simulink model "model1"  (R2024b)
settings: Solver=VariableStepAuto  StartTime=0.0  StopTime=10.0  RelTol=1e-3
libraries: simulink x4
settings Model: Creator=mehmetcanevi  LastModifiedBy=mehmetcanevi

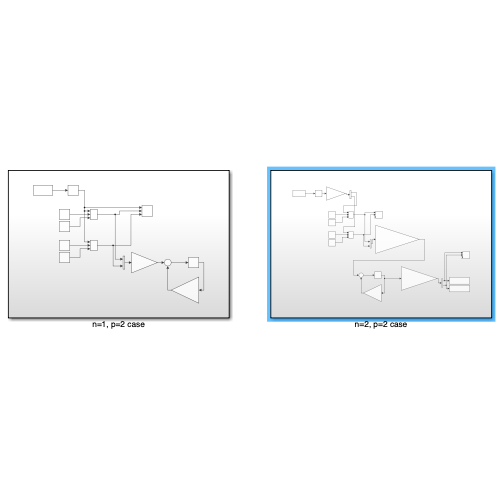
[thumbnail: Simulink's stored preview of the top-level diagram]
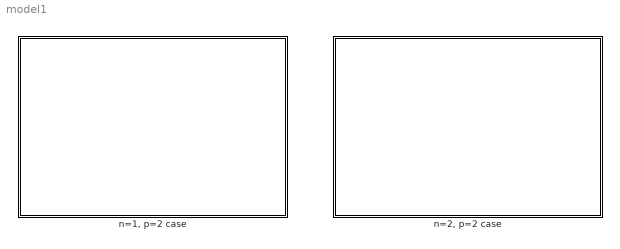
== system model1 ==
  "n=1, p=2 case" : Subsystem
  "n=2, p=2 case" : Subsystem

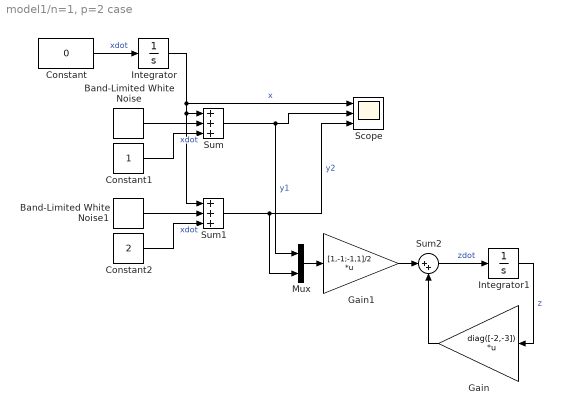
== system model1/n=1, p=2 case ==
  Band-Limited White Noise : simulink/Sources/Band-Limited White Noise  Cov=[0.001]  Ts=0.1  seed=[12345]
  Band-Limited White Noise1 : simulink/Sources/Band-Limited White Noise  Cov=[0.001]  Ts=0.1  seed=[12346]
  Constant : Constant  Value=0
  Constant1 : Constant
  Constant2 : Constant  Value=2
  Gain : Gain  Gain=diag([-2,-3])  Multiplication=Matrix(K*u)
  Gain1 : Gain  Gain=[1,-1;-1,1]/2  Multiplication=Matrix(K*u)
  Integrator : Integrator  InitialCondition=5
  Integrator1 : Integrator  InitialCondition=5
  Mux : Mux  Inputs=2
  Scope : Scope  NumInputPorts=3
  Sum : Sum  Inputs=+++
  Sum1 : Sum  Inputs=+++
  Sum2 : Sum  Inputs=|++
  wires:
  Sum2/1 -> Integrator1/1  "zdot"
  Constant1/1 -> Sum/3  "xdot"
  Band-Limited White Noise1/1 -> Sum1/2
  Integrator1/1 -> Gain/1  "z"
  Gain/1 -> Sum2/2
  Constant/1 -> Integrator/1  "xdot"
  Band-Limited White Noise/1 -> Sum/2
  Constant2/1 -> Sum1/3  "xdot"
  Integrator/1 -> Sum1/1, Sum/1, Scope/1  "x"
  Mux/1 -> Gain1/1
  Sum/1 -> Mux/1, Scope/2  "y1"
  Gain1/1 -> Sum2/1
  Sum1/1 -> Mux/2, Scope/3  "y2"

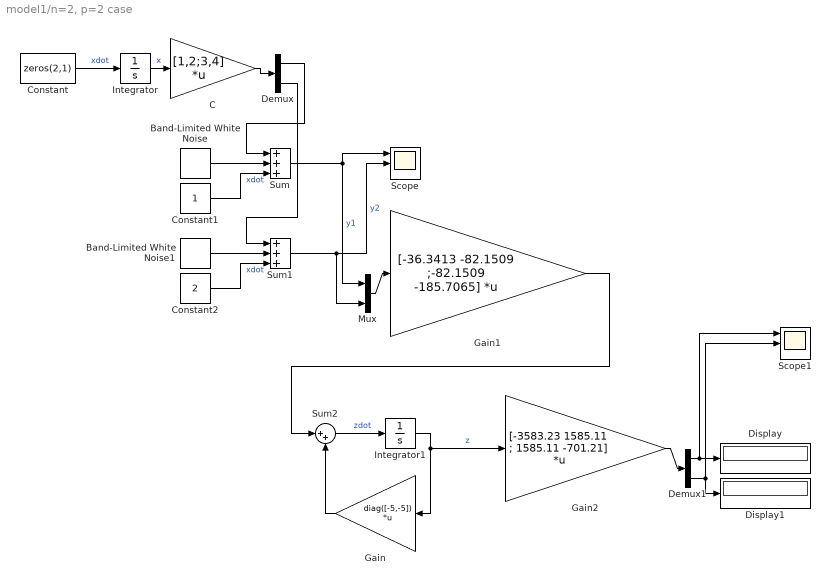
== system model1/n=2, p=2 case ==
  Band-Limited White Noise : simulink/Sources/Band-Limited White Noise  Cov=[0.001]  Ts=0.1  seed=[12345]
  Band-Limited White Noise1 : simulink/Sources/Band-Limited White Noise  Cov=[0.001]  Ts=0.1  seed=[12346]
  C : Gain  Gain=[1,2;3,4]  Multiplication=Matrix(K*u)
  Constant : Constant  Value=zeros(2,1)
  Constant1 : Constant
  Constant2 : Constant  Value=2
  Demux : Demux  Outputs=2
  Demux1 : Demux  Outputs=2
  Display : Display
  Display1 : Display
  Gain : Gain  Gain=diag([-5,-5])  Multiplication=Matrix(K*u)
  Gain1 : Gain  Gain=|  Multiplication=Matrix(K*u)
      | [-36.3413  -82.1509
      | ;-82.1509 -185.7065]
  Gain2 : Gain  Gain=|  Multiplication=Matrix(K*u)
      | [-3583.23       1585.11
      | ; 1585.11       -701.21]
  Integrator : Integrator  InitialCondition=[2;3]
  Integrator1 : Integrator  InitialCondition=5
  Mux : Mux  Inputs=2
  Scope : Scope  NumInputPorts=3
  Scope1 : Scope  NumInputPorts=3
  Sum : Sum  Inputs=+++
  Sum1 : Sum  Inputs=+++
  Sum2 : Sum  Inputs=|++
  wires:
  Sum2/1 -> Integrator1/1  "zdot"
  Constant1/1 -> Sum/3  "xdot"
  Band-Limited White Noise1/1 -> Sum1/2
  Integrator1/1 -> Gain/1, Gain2/1  "z"
  Gain/1 -> Sum2/2
  Constant/1 -> Integrator/1  "xdot"
  Band-Limited White Noise/1 -> Sum/2
  Constant2/1 -> Sum1/3  "xdot"
  Mux/1 -> Gain1/1
  Sum/1 -> Scope/1, Mux/1  "y1"
  Gain1/1 -> Sum2/1
  Sum1/1 -> Scope/2, Mux/2  "y2"
  Integrator/1 -> C/1  "x"
  C/1 -> Demux/1
  Demux/1 -> Sum/1
  Demux/2 -> Sum1/1
  Gain2/1 -> Demux1/1
  Demux1/1 -> Scope1/1, Display/1
  Demux1/2 -> Display1/1, Scope1/2
